simulink model "ode_solver_3d"  (R2023a)
settings: Solver=VariableStepAuto  StartTime=0.0  StopTime=10.0  RelTol=1e-3
settings Model: Creator=joaog  LastModifiedBy=joaog

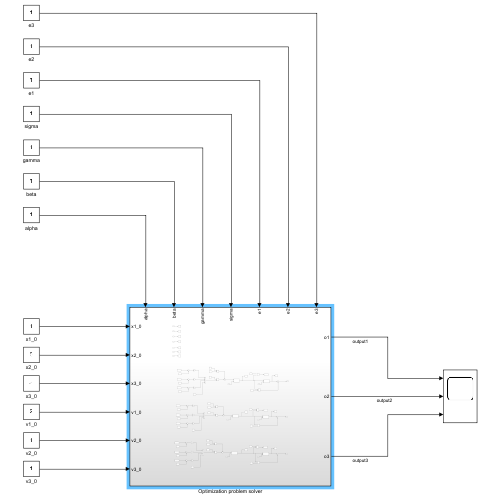
[thumbnail: Simulink's stored preview of the top-level diagram]
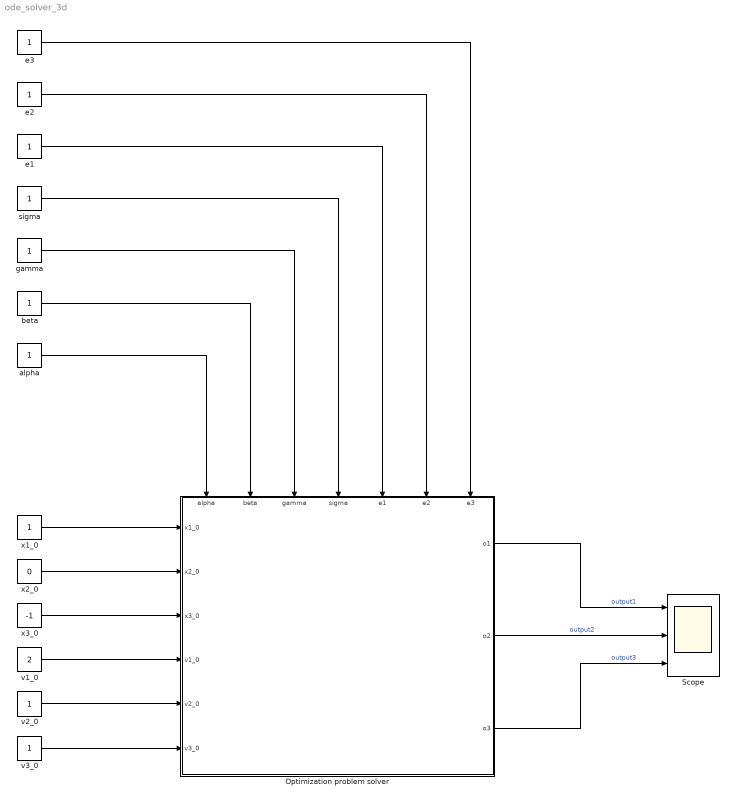
== system ode_solver_3d ==
  Optimization problem solver : Subsystem
      settings: PortSchema="{\"entries\":[{\"content\":{\"sides\":[{\"content\":{\"connectorIds\":[\"In1\",\"In2\",\"In3\",\"In4\",\"In5\",\"In6\"]},\"type\":\"ConnectorPlacement.EquallySpacedRectSide\",\"uuid\":\"ace58a2b-4bbe-49a2-915d-fce3e7b8fef9\"},{\"content\":{\"connectorIds\":[\"Out1\",\"Out2\",\"Out3\"],\"side\":\"RIGHT\"},\"type\":\"ConnectorPlacement.EquallySpacedRectSide\",\"uuid\":\"d7f2c16b-5f0e-4f62-a2af-5253be17176a\"},{\"content\":{\"connectorIds\":[\"In7\",\"In8\",\"In9\",\"In10\",\"In11\",\"In12\",\"In13\"],\"side\":\"TOP\"},\"type\":\"ConnectorPlacement.EquallySpacedRectSide\",\"uuid\":\"f696cb1b-8c75-4876-acf7-079715f4e536\"}]},\"type\":\"ConnectorPlacement.EquallySpacedConnector\",\"uuid\":\"3d890d1a-9284-4c35-bb22-db42113889f5\"}],\"packageUris\":[\"http://schema.mathworks.com/mf0/Connector/R2020b\"],\"version\":\"1.0\"}"
  Scope : Scope  NumInputPorts=3
  alpha : Constant
  beta : Constant
  e1 : Constant
  e2 : Constant
  e3 : Constant
  gamma : Constant
  sigma : Constant
  v1_0 : Constant  Value=2
  v2_0 : Constant
  v3_0 : Constant
  x1_0 : Constant
  x2_0 : Constant  Value=0
  x3_0 : Constant  Value=-1
  wires:
  alpha/1 -> Optimization problem solver/7(alpha)
  beta/1 -> Optimization problem solver/8(beta)
  gamma/1 -> Optimization problem solver/9(gamma)
  sigma/1 -> Optimization problem solver/10(sigma)
  e1/1 -> Optimization problem solver/11(e1)
  e2/1 -> Optimization problem solver/12(e2)
  e3/1 -> Optimization problem solver/13(e3)
  x1_0/1 -> Optimization problem solver/1(x1_0)
  x2_0/1 -> Optimization problem solver/2(x2_0)
  x3_0/1 -> Optimization problem solver/3(x3_0)
  v1_0/1 -> Optimization problem solver/4(v1_0)
  v2_0/1 -> Optimization problem solver/5(v2_0)
  v3_0/1 -> Optimization problem solver/6(v3_0)
  Optimization problem solver/1(o1) -> Scope/1  "output1"
  Optimization problem solver/2(o2) -> Scope/2  "output2"
  Optimization problem solver/3(o3) -> Scope/3  "output3"

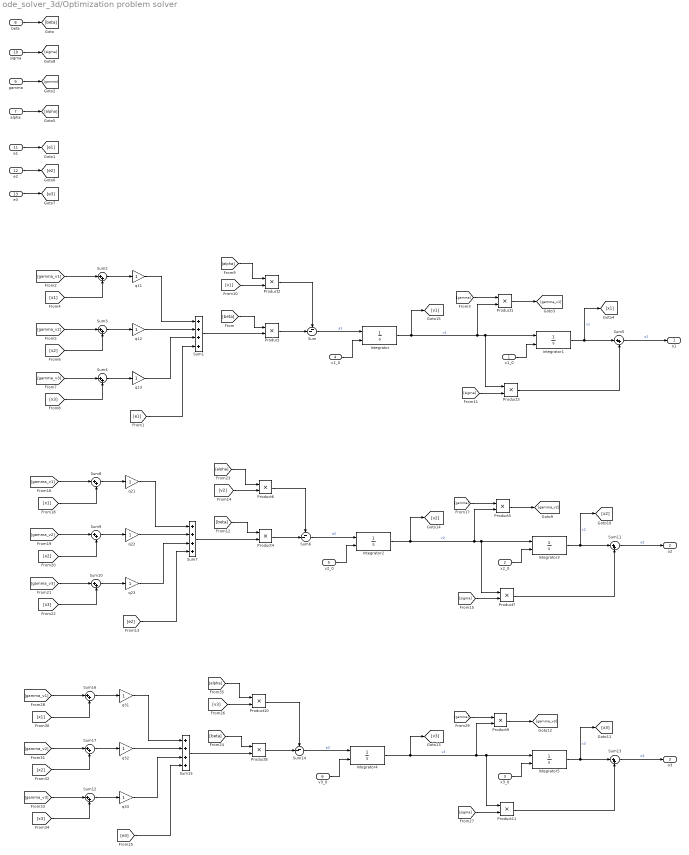
== system ode_solver_3d/Optimization problem solver ==
  x1_0 : Inport
  x2_0 : Inport  Port=2
  x3_0 : Inport  Port=3
  v1_0 : Inport  Port=4
  v2_0 : Inport  Port=5
  v3_0 : Inport  Port=6
  alpha : Inport  Port=7
  beta : Inport  Port=8
  gamma : Inport  Port=9
  sigma : Inport  Port=10
  e1 : Inport  Port=11
  e2 : Inport  Port=12
  e3 : Inport  Port=13
  Integrator{,1..5} (6 alike) : Integrator  InitialConditionSource=external
  Product{,1..11} (12 alike) : Product
  Sum : Sum  Inputs=--|
  Sum1 : Sum  Inputs=++++
  Sum{2..5,8..13,16..17} (12 alike) : Sum  Inputs=|++
  Sum14 : Sum  Inputs=--|
  Sum15 : Sum  Inputs=++++
  Sum6 : Sum  Inputs=--|
  Sum7 : Sum  Inputs=++++
  q{11..13,21..23,31..33} (9 alike) : Gain
  o1 : Outport
  o2 : Outport  Port=2
  o3 : Outport  Port=3
  wires:
  [gamma_v1] -> Sum8/1
  Sum8/1 -> q21/1
  q31/1 -> Sum15/1
  Integrator/1 -> [v1], Integrator1/1, Product3/1, Product1/2  "v1"
  Integrator4/1 -> [v3], Integrator5/1, Product11/1, Product9/2  "v3"
  Product7/1 -> Sum11/2
  Integrator5/1 -> [x3], Sum13/1  "x3"
  q12/1 -> Sum1/2
  Integrator3/1 -> [x2], Sum11/1  "x2"
  Sum10/1 -> q23/1
  [gamma_v2] -> Sum9/1
  [beta] -> Product4/1
  Sum1/1 -> Product/2
  [beta] -> Product/1
  Sum7/1 -> Product4/2
  sigma/1 -> [sigma]
  Product/1 -> Sum/2
  Integrator2/1 -> [v2], Product5/2, Integrator3/1, Product7/1  "v2"
  [e1] -> Sum1/4
  Sum14/1 -> Integrator4/1  "a3"
  [gamma_v1] -> Sum2/1
  Sum9/1 -> q22/1
  Sum5/1 -> o1/1  "o1"
  q21/1 -> Sum7/1
  beta/1 -> [beta]
  Product1/1 -> [gamma_v1]
  [x2] -> Sum9/2
  Sum3/1 -> q12/1
  e1/1 -> [e1]
  [x3] -> Sum10/2
  Product3/1 -> Sum5/2
  [beta] -> Product8/1
  [alpha] -> Product6/1
  e2/1 -> [e2]
  Sum/1 -> Integrator/1  "a1"
  Integrator1/1 -> [x1], Sum5/1  "x1"
  Product5/1 -> [gamma_v2]
  Sum6/1 -> Integrator2/1  "a2"
  [alpha] -> Product2/1
  x1_0/1 -> Integrator1/2
  Sum4/1 -> q13/1
  q11/1 -> Sum1/1
  e3/1 -> [e3]
  [v2] -> Product6/2
  Product11/1 -> Sum13/2
  Product4/1 -> Sum6/2
  Product6/1 -> Sum6/1
  Sum11/1 -> o2/1  "o2"
  [gamma_v3] -> Sum10/1
  [x1] -> Sum2/2
  v2_0/1 -> Integrator2/2
  Sum16/1 -> q31/1
  x2_0/1 -> Integrator3/2
  q23/1 -> Sum7/3
  [x1] -> Sum8/2
  alpha/1 -> [alpha]
  [gamma_v2] -> Sum3/1
  [gamma] -> Product5/1
  [gamma] -> Product1/1
  [sigma] -> Product7/2
  [gamma_v3] -> Sum4/1
  q22/1 -> Sum7/2
  q13/1 -> Sum1/3
  [e2] -> Sum7/4
  [e3] -> Sum15/4
  Sum12/1 -> q33/1
  [x2] -> Sum3/2
  Sum2/1 -> q11/1
  gamma/1 -> [gamma]
  [sigma] -> Product3/2
  [x3] -> Sum4/2
  Product2/1 -> Sum/1
  [v1] -> Product2/2
  v1_0/1 -> Integrator/2
  [v3] -> Product10/2
  [gamma] -> Product9/1
  [x1] -> Sum16/2
  q32/1 -> Sum15/2
  Product10/1 -> Sum14/1
  [sigma] -> Product11/2
  Sum17/1 -> q32/1
  Product9/1 -> [gamma_v3]
  [x2] -> Sum17/2
  [x3] -> Sum12/2
  x3_0/1 -> Integrator5/2
  Sum15/1 -> Product8/2
  [gamma_v2] -> Sum17/1
  q33/1 -> Sum15/3
  [alpha] -> Product10/1
  [gamma_v3] -> Sum12/1
  Sum13/1 -> o3/1  "o3"
  Product8/1 -> Sum14/2
  v3_0/1 -> Integrator4/2
  [gamma_v1] -> Sum16/1
